simulink model "Kalmant"  (R2021b)
settings: Solver=FixedStepAuto  StartTime=0.0  StopTime=200  FixedStep=1e-4  RelTol=1e-3
libraries: commchan3 x1, spspowerguiLib x1
settings Model: Creator=12406  LastModifiedBy=aryal
settings SolverCC: AlgebraicLoopSolver=TrustRegion

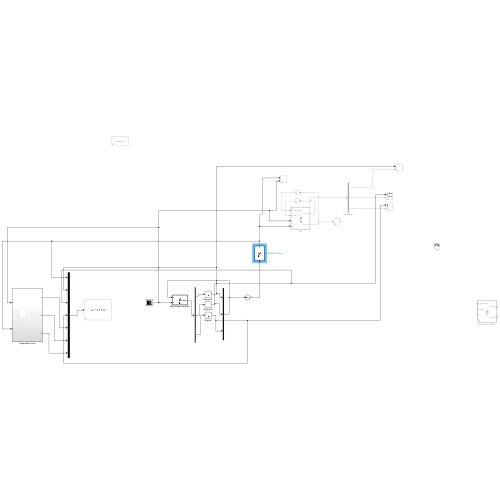
[thumbnail: Simulink's stored preview of the top-level diagram]
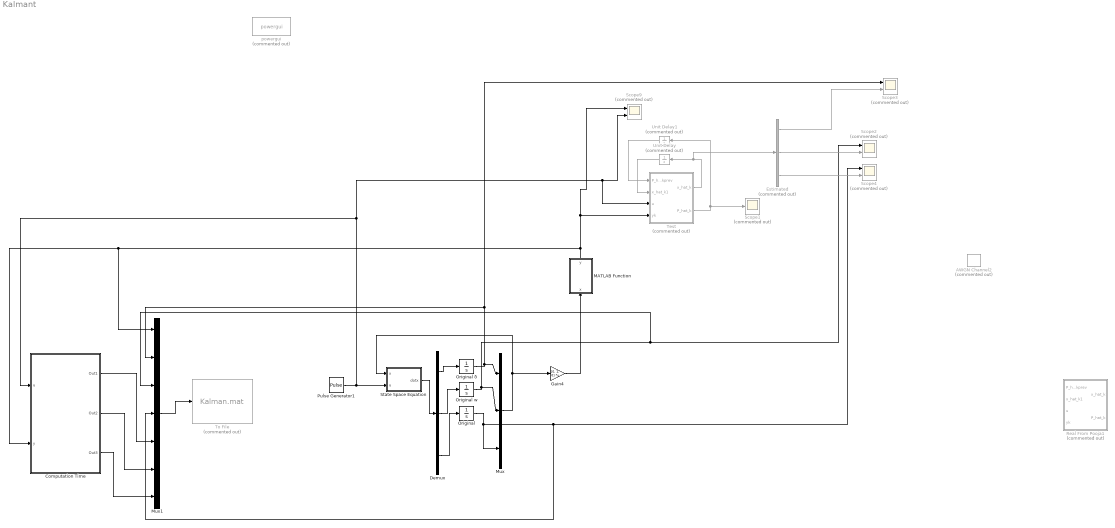
== system Kalmant ==
  AWGN Channel2 : commchan3/AWGN Channel  Commented=on  InputProcessing=Columns as channels (frame based)  seed=65  noiseMode=Variance from mask  EbNodB=10  EsNodB=10  SNRdB=65  bitsPerSym=1  Ps=1  Tsym=1  variance=1e-6
  Computation Time : Subsystem
  Demux : Demux  Outputs=3
  Estimated : Demux  Commented=on  Outputs=3
  Gain4 : Gain  Gain=[0, 1, 0]  Multiplication=Matrix(K*u)
  MATLAB Function : MATLAB Function  TreatAsAtomicUnit=on
  Mux : Mux  Inputs=3
  Mux1 : Mux  Inputs=7
  "Original " : Integrator
  Original w : Integrator
  "Original δ " : Integrator
  Pulse Generator1 : DiscretePulseGenerator  PulseType=Time based  Amplitude=0.2  PulseWidth=50
  Real From Pooja1 : MATLAB Function  Commented=on  TreatAsAtomicUnit=on  SystemSampleTime=0.02
  Scope1 : Scope  Commented=on
  Scope{2..4,9} (4 alike) : Scope  Commented=on  NumInputPorts=2
  State Space Equation : MATLAB Function  TreatAsAtomicUnit=on
  Test : MATLAB Function  Commented=on  TreatAsAtomicUnit=on  SystemSampleTime=0.02
  To File : ToFile  Commented=on  Filename=Kalman.mat  MatrixName=w  SampleTime=0.02
  Unit Delay : UnitDelay  Commented=on  InitialCondition=zeros(3, 1)  SampleTime=0.02  HasFrameUpgradeWarning=on
  Unit Delay1 : UnitDelay  Commented=on  InitialCondition=ones(9, 1)*100  SampleTime=0.02  HasFrameUpgradeWarning=on
  powergui : spspowerguiLib/powergui  Priority=1  Commented=on  SimulationMode=Continuous  SampleTime=50e-6  frequency=60  Iterations=50  frequencyindice=0  Pbase=100e6  ErrMax=1e-4  UnitsV=kV  UnitsW=MW  buscounter=0  FunctionMessages=off  echomessages=off  EnableUseOfTLC=off  CurrentSourceSwitches=off  DisableSnubberDevices=off  DisableRonSwitches=off  DisableVfSwitches=off  DisplayEquations=off  AutomaticDiscreteSolvers=off  SolverType=Tustin/Backward Euler (TBE)  Interpol=off  ExternalGateDelay=off  methode=off  Ts=100  x0status=blocks  SPID=on  SwTol=0  HookPort=off  NonlinearTolerance=1e-4  nMaxIteration=100  ContinueOnMaxIteration=off  RestoreLinks=warning  ResistiveCurrentMeasurement=off  Frange=[0:2:500]  Ylog=off  Xlog=on  ShowGrid=off  save=off  variable=ZData  structure=0  ZoomFFT=off  StartTime=0.0  cycles=1  DisplayStyle=1  fundamental=60  FreqAxis=off  MaxFrequency=1000  frequencyindicesteady=1  RmsSteady=1  display=off
  wires:
  Mux/1 -> Gain4/1, State Space Equation/1(x)
  Gain4/1 -> MATLAB Function/1(x)
  Pulse Generator1/1 -> Test/3(u), Scope9/2, Computation Time/1(u), State Space Equation/2(u)
  Original w/1 -> Mux1/3, Scope2/1, Mux/2
  Demux/2 -> Original w/1
  Demux/1 -> "Original δ "/1
  "Original δ "/1 -> Scope3/1, Mux1/2, Mux/1
  State Space Equation/1(dotx) -> Demux/1
  Demux/3 -> "Original "/1
  "Original "/1 -> Mux1/4, Scope4/1, Mux/3
  MATLAB Function/1(y) -> Test/4(yk), Scope9/1, Mux1/1, Computation Time/2(y)
  Test/1(x_hat_k) -> Estimated/1, Unit Delay/1
  Test/2(P_hat_k) -> Unit Delay1/1, Scope1/1
  Unit Delay1/1 -> Test/1(P_hat_kprev)
  Estimated/1 -> Scope3/2
  Estimated/2 -> Scope2/2
  Estimated/3 -> Scope4/2
  Unit Delay/1 -> Test/2(x_hat_k1)
  Computation Time/1(Out1) -> Mux1/5
  Computation Time/2(Out2) -> Mux1/6
  Computation Time/3(Out3) -> Mux1/7
  Mux1/1 -> To File/1

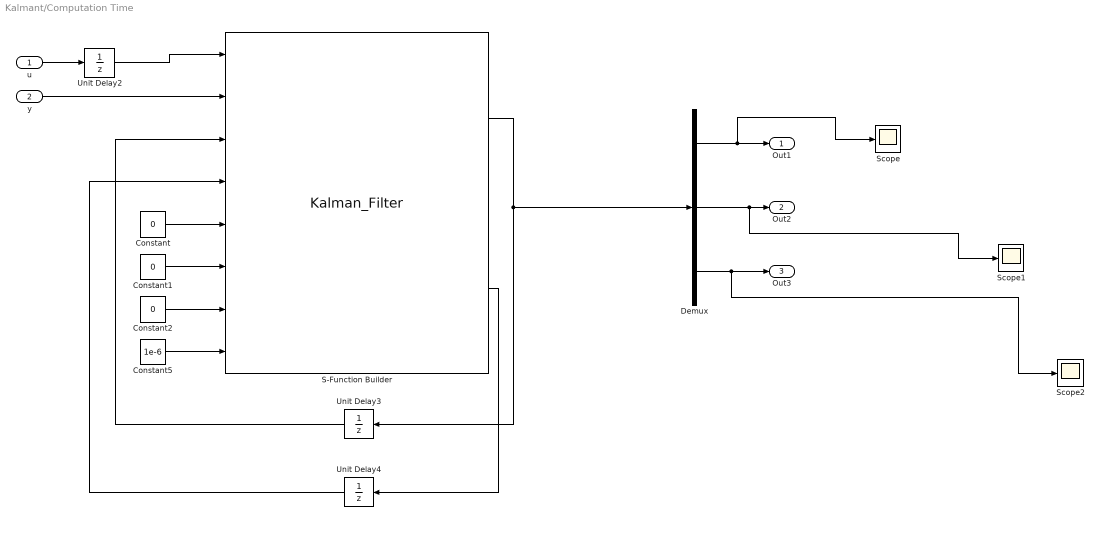
== system Kalmant/Computation Time ==
  u : Inport
  y : Inport  Port=2
  Constant : Constant  Value=0
  Constant1 : Constant  Value=0
  Constant2 : Constant  Value=0
  Constant5 : Constant  Value=1e-6
  Demux : Demux  Outputs=3
  S-Function Builder : S-Function  FunctionName=Kalman_Filter  SFunctionModules=Kalman_Filter_wrapper KF_Code KF_Code_Call  SFunctionDeploymentMode=off  EnableBusSupport=off  mask(S-Function Builder){}
      mask help: Simulink:masks:SFunctionBuilder_MD
      mask init:
      | val = [[.9  0.75 0.75 1 1 .9 .9 1]',[1 1 0.75 0.75 .9 .9 1 .9]'];try , sys = get_param(gcb,'SfunBuilderFcnName');if isempty(sys), sys = get_param(gcb,'FunctionName'); end,catch, sys = get_param(gcb,'FunctionName'); end
      settings: CopyFcn=set_param(gcbh,'LinkStatus','none')  OpenFcn=sfunctionwizard(gcbh)
      mask Display:
      | plot(val(:,1),val(:,2))
      | disp(sys)
      | port_label('input',1,'u')
      | port_label('input',2,'y')
      | port_label('input',3,'xhatp')
      | port_label('input',4,'Pkp')
      | port_label('input',5,'Q11')
      | port_label('input',6,'Q22')
      | port_label('input',7,'Q33')
      | port_label('input',8,'R')
      | port_label('output',1,'xhat')
      | port_label('output',2,'Pk')
  Scope : Scope
  Scope1 : Scope
  Scope2 : Scope
  Unit Delay2 : UnitDelay  SampleTime=0.02  HasFrameUpgradeWarning=on
  Unit Delay3 : UnitDelay  InitialCondition=[0;0;0]  SampleTime=0.02  HasFrameUpgradeWarning=on
  Unit Delay4 : UnitDelay  InitialCondition=reshape(diag([10, 10, 10]), 9, 1)  SampleTime=0.02  HasFrameUpgradeWarning=on
  Out1 : Outport
  Out2 : Outport  Port=2
  Out3 : Outport  Port=3
  wires:
  Unit Delay4/1 -> S-Function Builder/4
  Unit Delay3/1 -> S-Function Builder/3
  u/1 -> Unit Delay2/1
  Constant/1 -> S-Function Builder/5
  Constant5/1 -> S-Function Builder/8
  Constant2/1 -> S-Function Builder/7
  S-Function Builder/1 -> Demux/1, Unit Delay3/1
  y/1 -> S-Function Builder/2
  Constant1/1 -> S-Function Builder/6
  S-Function Builder/2 -> Unit Delay4/1
  Unit Delay2/1 -> S-Function Builder/1
  Demux/1 -> Scope/1, Out1/1
  Demux/2 -> Scope1/1, Out2/1
  Demux/3 -> Scope2/1, Out3/1

== matlab function Kalmant/MATLAB Function ==
  data: x input; y output
function y = fcn(x)

y = x + pearsrnd(0, 1e-3, -0.5, 7.0);

== matlab function Kalmant/State Space Equation ==
  data: x input; u input; dotx output
function dotx  = fcn(x, u)
D = 1.5;
M = 4.0;
    Tg = 0.2;
    Rp = 0.05;
    Ki=2;
    dotx = zeros(3, 1);
    x1 = x(1);
    x2 = x(2);
    x3=x(3);
    dotx = [x2;x3;-Ki/(M*Tg)*x1-(D/(M*Tg)+1/(Rp*M*Tg))*x2-(D/M+1/Tg)*x3-1/(M*Tg)*u];

== matlab function Kalmant/Test ==
  data: P_hat_kprev input; x_hat_k1 input; u input; x_hat_k output; P_hat_k output; yk input
function [x_hat_k,P_hat_k] = fcn(P_hat_kprev, x_hat_k1,u,yk)
 M=4;
 ki=2;
 Tg=0.2;
 Rp=0.05;
 D=1.5;
A= [1.0000    0.0200    0.0002;
   -0.0005    0.9948    0.0189;
   -0.0473   -0.5092    0.8931];
B=[-0.0000;
   -0.0002;
   -0.0237];
P_hat_k1 = reshape(P_hat_kprev, [3, 3]);
p_hat_k = zeros(9,1);
x_hat_k = zeros(3, 1);

C=[0,1,0];
%covaraince initialize
R = 1e-6;
Q = eye(3,3)*1e-7;
%Prediction step

xp_hat_k=A*x_hat_k1+B*u;
Pp=A*P_hat_k1*A'+Q;

%Update step
kf=(Pp*C')/(C*Pp*C'+R);
x_hat_k=xp_hat_k+kf*(yk-C*xp_hat_k);
P_hat_k=reshape((eye(3)-kf*C)*Pp, [9, 1]);

== matlab function Kalmant/Real From Pooja1 ==
  data: P_hat_kprev input; x_hat_k1 input; u input; x_hat_k output; P_hat_k output; yk input
function [x_hat_k,P_hat_k] = fcn(P_hat_kprev, x_hat_k1,u,yk)
 M=4;
 ki=2;
 Tg=0.2;
 Rp=0.05;
 D=0.015;
A= [0.999967500625000   0.019967309583802   0.000193328458427;

  -0.004833211460677   0.995130664255727   0.018999942309948;

  -0.474998557748689  -0.480188018127678   0.900059702922327];
B=[-0.000001624968750;

  -0.000241660573034;

  -0.023749927887434];
P_hat_k1 = reshape(P_hat_kprev, [3, 3]);
p_hat_k = zeros(9,1);
x_hat_k = zeros(3, 1);

C=[0,1,0];
%covaraince initialize
R = 1e-6;
Q = eye(3,3)*1e-7;
%Prediction step

xp_hat_k=A*x_hat_k1+B*u;
Pp=A*P_hat_k1*A'+Q;

%Update step
kf=(Pp*C')/(C*Pp*C'+R);
x_hat_k=xp_hat_k+kf*(yk-C*xp_hat_k);
P_hat_k=reshape((eye(3)-kf*C)*Pp, [9, 1]);
